simulink library "controllerUDPNode_ul"  (R2018b)
settings: Solver=VariableStepAuto  StartTime=0.0  StopTime=10.0  RelTol=1e-3
undefined symbols (not defined in the file): ipaddr, PTP
libraries: xpcutilitieslib x6, xpcrtudplib x6, ptplib x3
settings Model: Creator=MAE-NCSUCORE  LastModifiedBy=MAE-NCSUCORE

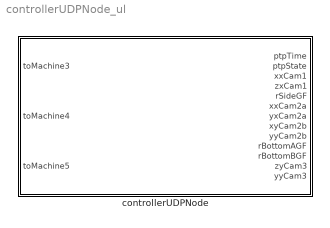
== system controllerUDPNode_ul ==
  controllerUDPNode : Subsystem  TreatAsAtomicUnit=on  mask{annouceInterval=1, syncInterval=0.05}
      mask prompts: annouceInterval "Announce Interval [s]"; syncInterval "Sync Interval [s]"

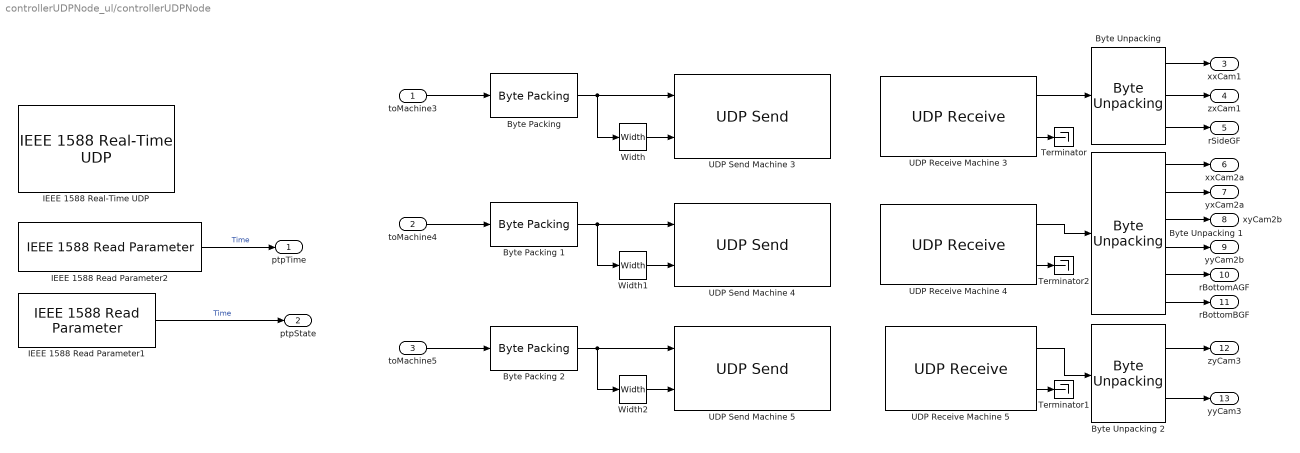
== system controllerUDPNode_ul/controllerUDPNode ==
  toMachine3 : Inport
  toMachine4 : Inport  Port=2
  toMachine5 : Inport  Port=3
  "Byte Packing " : xpcutilitieslib/Byte Packing   MaskPackedDataType=uint8  MaskUnpackedDataTypes={['uint8']}  MaskAlignment=1
  Byte Packing 1 : xpcutilitieslib/Byte Packing   MaskPackedDataType=uint8  MaskUnpackedDataTypes={['uint8']}  MaskAlignment=1
  Byte Packing 2 : xpcutilitieslib/Byte Packing   MaskPackedDataType=uint8  MaskUnpackedDataTypes={['uint8']}  MaskAlignment=1
  "Byte Unpacking " : xpcutilitieslib/Byte Unpacking   MaskUnpackedDataTypes={'double','double',['uint8']}  MaskUnpackedDataSizes={[1],[1],[3]}  MaskAlignment=1
      settings: SourceProductName=Simulink Real-Time  SourceProductBaseCode=XP
  Byte Unpacking 1 : xpcutilitieslib/Byte Unpacking   MaskUnpackedDataTypes={'double','double','double','double',['uint8'],['uint8']}  MaskUnpackedDataSizes={[1],[1],[1],[1],[3],[3]}  MaskAlignment=1
      settings: SourceProductName=Simulink Real-Time  SourceProductBaseCode=XP
  Byte Unpacking 2 : xpcutilitieslib/Byte Unpacking   MaskUnpackedDataTypes={'double','double'}  MaskUnpackedDataSizes={[1],[1]}  MaskAlignment=1
      settings: SourceProductName=Simulink Real-Time  SourceProductBaseCode=XP
  IEEE 1588 Read Parameter1 : ptplib/IEEE 1588 Read Parameter  Priority=1  ID=1  param=Protocol state  sample_time=0.01  enable_read_precision=off
      settings: SourceProductName=Simulink Real-Time  SourceProductBaseCode=XP
  IEEE 1588 Read Parameter2 : ptplib/IEEE 1588 Read Parameter  Priority=1  ID=1  param=PTP time (time-of-day)  sample_time=0.01  enable_read_precision=off
      settings: SourceProductName=Simulink Real-Time  SourceProductBaseCode=XP
  IEEE 1588 Real-Time UDP : ptplib/IEEE 1588 Real-Time UDP  Priority=0  ID=1  PciBus=2  PciSlot=0  PciFunction=0  time_inc=4000000  sample_time=0.01  IpSource=Specify  IpAddress=30.30.30.30  SubnetMask=255.255.255.0  Gateway=0.0.0.0  Receive1=0.0.0.0  dest_ip_select=Specify  custom_dest_ip_addr=255.255.255.255  MulticastList=[ipaddr('224.0.1.129'), ipaddr('224.0.0.107')]  Multicast={macaddr('01:00:5E:00:01:81'), macaddr('01:00:5E:00:00:6B')}  time_source=Ethernet board  timescale=PTP (1970-01-01)  epoch=[1970 01 01 00]  delay_measure=Request-response  slave_only=off  enable_advanced_config=on  domain_num=0  utc_offset=35  priority1=1  clock_class=248  clock_accuracy=hex2dec('FE')  priority2=1  announce_interval=announceInterval  sync_interval=syncInterval  min_pdelay_req_interval=0.1  announce_receipt_timeout=3
      settings: SourceProductName=Simulink Real-Time  SourceProductBaseCode=XP
  Terminator : Terminator
  Terminator1 : Terminator
  Terminator2 : Terminator
  UDP Receive Machine 3 : xpcrtudplib/UDP Receive  ipAddressVal=30.30.30.30  localPort=8001  rcvWidth=8  rcvFmAny=off  fmAddress=30.30.30.1  rcvMulticast=off  multicastAddress={30.30.30.1, 30.30.30.2, 30.30.30.3}  maxUDPQueue=8  sampleTime=0.01
      settings: SourceProductName=Simulink Real-Time
  UDP Receive Machine 4 : xpcrtudplib/UDP Receive  ipAddressVal=30.30.30.30  localPort=8002  rcvWidth=8  rcvFmAny=off  fmAddress=30.30.30.2  rcvMulticast=off  multicastAddress={30.30.30.1, 30.30.30.2, 30.30.30.3}  maxUDPQueue=8  sampleTime=0.01
      settings: SourceProductName=Simulink Real-Time
  UDP Receive Machine 5 : xpcrtudplib/UDP Receive  ipAddressVal=30.30.30.30  localPort=8003  rcvWidth=8  rcvFmAny=off  fmAddress=30.30.30.3  rcvMulticast=off  multicastAddress={30.30.30.1, 30.30.30.2, 30.30.30.3}  maxUDPQueue=8  sampleTime=0.01
      settings: SourceProductName=Simulink Real-Time
  UDP Send Machine 3 : xpcrtudplib/UDP Send  ipAddressVal=30.30.30.30  localPort=8001  toAddress=30.30.30.1  toPort=8000  sampleTime=0.01
      settings: SourceProductName=Simulink Real-Time  SourceProductBaseCode=XP
  UDP Send Machine 4 : xpcrtudplib/UDP Send  ipAddressVal=30.30.30.30  localPort=8002  toAddress=30.30.30.2  toPort=8000  sampleTime=0.01
      settings: SourceProductName=Simulink Real-Time  SourceProductBaseCode=XP
  UDP Send Machine 5 : xpcrtudplib/UDP Send  ipAddressVal=30.30.30.30  localPort=8003  toAddress=30.30.30.3  toPort=8000  sampleTime=0.01
      settings: SourceProductName=Simulink Real-Time  SourceProductBaseCode=XP
  Width : Width
  Width1 : Width
  Width2 : Width
  ptpTime : Outport
  ptpState : Outport  Port=2
  xxCam1 : Outport  Port=3
  zxCam1 : Outport  Port=4
  rSideGF : Outport  Port=5
  xxCam2a : Outport  Port=6
  yxCam2a : Outport  Port=7
  xyCam2b : Outport  Port=8
  yyCam2b : Outport  Port=9
  rBottomAGF : Outport  Port=10
  rBottomBGF : Outport  Port=11
  zyCam3 : Outport  Port=12
  yyCam3 : Outport  Port=13
  wires:
  UDP Receive Machine 4/2 -> Terminator2/1
  "Byte Packing "/1 -> Width/1, UDP Send Machine 3/1
  Width/1 -> UDP Send Machine 3/2
  Width1/1 -> UDP Send Machine 4/2
  UDP Receive Machine 3/2 -> Terminator/1
  Width2/1 -> UDP Send Machine 5/2
  IEEE 1588 Read Parameter2/1 -> ptpTime/1  "Time"
  UDP Receive Machine 3/1 -> "Byte Unpacking "/1
  UDP Receive Machine 4/1 -> Byte Unpacking 1/1
  Byte Packing 1/1 -> Width1/1, UDP Send Machine 4/1
  Byte Packing 2/1 -> Width2/1, UDP Send Machine 5/1
  UDP Receive Machine 5/2 -> Terminator1/1
  toMachine3/1 -> "Byte Packing "/1
  toMachine5/1 -> Byte Packing 2/1
  toMachine4/1 -> Byte Packing 1/1
  "Byte Unpacking "/1 -> xxCam1/1
  Byte Unpacking 2/1 -> zyCam3/1
  IEEE 1588 Read Parameter1/1 -> ptpState/1  "Time"
  "Byte Unpacking "/2 -> zxCam1/1
  "Byte Unpacking "/3 -> rSideGF/1
  Byte Unpacking 1/1 -> xxCam2a/1
  Byte Unpacking 1/2 -> yxCam2a/1
  Byte Unpacking 1/3 -> xyCam2b/1
  Byte Unpacking 1/4 -> yyCam2b/1
  Byte Unpacking 1/5 -> rBottomAGF/1
  Byte Unpacking 1/6 -> rBottomBGF/1
  UDP Receive Machine 5/1 -> Byte Unpacking 2/1
  Byte Unpacking 2/2 -> yyCam3/1
